simulink model "Pub_Sub_Husqvarna_Smartwatch"  (R2017a)
settings: Solver=VariableStepAuto  StartTime=0.0  StopTime=inf  RelTol=1e-3
undefined symbols (not defined in the file): Angular, Linear
libraries: robotlib x3, fuzblock x1
settings Model: Creator=francesco  LastModifiedBy=francesco

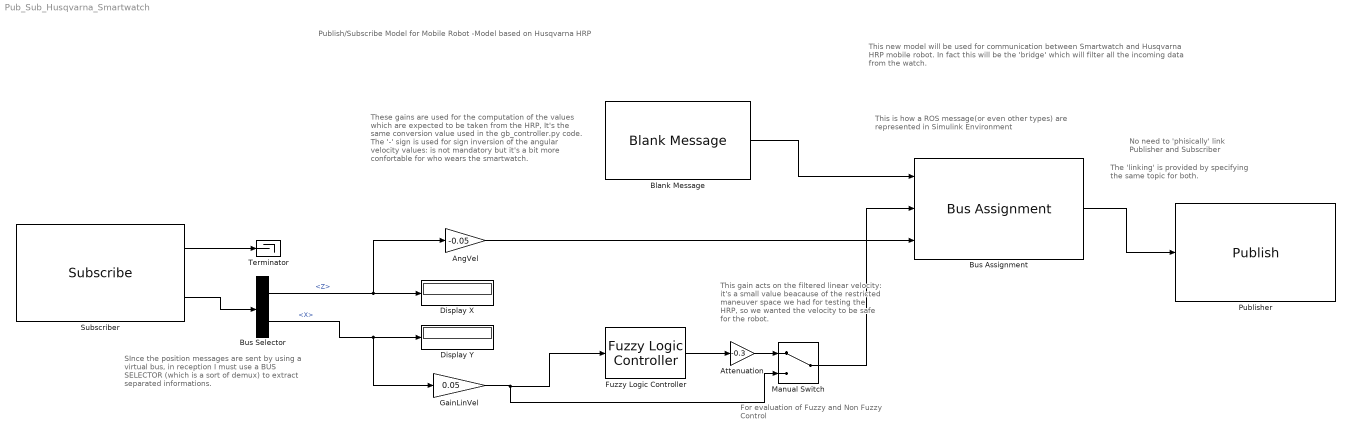
== system Pub_Sub_Husqvarna_Smartwatch ==
  note: This gain acts on the filtered linear
      | velocity: it's a small value beacause
      | of the restricted maneuver space we had
      | for testing the HRP, so we wanted the
      | velocity to be safe for the robot.
  note: These gains are used for the
      | computation of the values which are
      | expected to be taken from the HRP,
      | It's the same conversion value used in the
      | gb_controller.py code.
      | The '-' sign is used for sign inversion of the
      | angular velocity values: is not mandatory but
      | it's a bit more confortable for who wears the
      | smartwatch.
  note: This new model will be used for communication between Smartwatch and
      | Husqvarna HRP mobile robot.
      | In fact this will be the 'bridge' which will filter all the incoming data from the watch.
  note: Publish/Subscribe Model for Mobile Robot
      | -Model based on Husqvarna HRP
  note: The 'linking' is provided by specifying
      | the same topic for both.
  note: For evaluation of Fuzzy and Non Fuzzy
      | Control
  note: No need to 'phisically' link
      | Publisher and Subscriber
  note: This is how a ROS message(or even other types)
      |  are represented in Simulink Environment
  note: SInce the position messages are sent by
      | using a virtual bus, in reception I must use
      | a BUS SELECTOR (which is a sort of demux)
      |  to extract separated informations.
  AngVel : Gain  Gain=-0.05
  Attenuation : Gain  Gain=-0.3
  Blank Message : robotlib/Blank Message  SourceLibraryInfo=This block requires Robotics System Toolbox  messageType=geometry_msgs/Twist  SampleTime=inf
      settings: SourceProductBaseCode=RO
  Bus Assignment : BusAssignment  AssignedSignals=Linear.X,Angular.Z
  Bus Selector : BusSelector  OutputSignals=LinearAcceleration.Z,LinearAcceleration.X
  Display X : Display
  Display Y : Display
  Fuzzy Logic Controller : fuzblock/Fuzzy Logic  Controller  fis='LinVelDefinitivo.fis'
  GainLinVel : Gain  Gain=0.05
  Manual Switch : ManualSwitch
  Publisher : robotlib/Publish  SourceLibraryInfo=This block requires Robotics System Toolbox  topicSource=Select from ROS network  topic=/cmd_vel  messageType=geometry_msgs/Twist  messageQueueLength=1
      settings: SourceProductBaseCode=RO
  Subscriber : robotlib/Subscribe  SourceLibraryInfo=This block requires Robotics System Toolbox  topicSource=Select from ROS network  topic=/inertial  messageType=sensor_msgs/Imu  sampleTime=-1  messageQueueLength=1
      settings: SourceProductBaseCode=RO
  Terminator : Terminator
  wires:
  Attenuation/1 -> Manual Switch/1
  Bus Assignment/1 -> Publisher/1
  Fuzzy Logic Controller/1 -> Attenuation/1
  Blank Message/1 -> Bus Assignment/1
  Bus Selector/1 -> AngVel/1, Display X/1  "<Z>"
  Bus Selector/2 -> GainLinVel/1, Display Y/1  "<X>"
  Subscriber/1 -> Terminator/1
  Subscriber/2 -> Bus Selector/1
  Manual Switch/1 -> Bus Assignment/2
  AngVel/1 -> Bus Assignment/3
  GainLinVel/1 -> Manual Switch/2, Fuzzy Logic Controller/1
